simulink model "model_for_lab_2"  (R2022b)
settings: Solver=VariableStepAuto  StartTime=0.0  StopTime=1  RelTol=1e-3
values from neighbouring files (symbols this model uses):
  J = gear_ratio^2 * J_ed    (= 0.0023919264)    [m_for_lab_2.m]
  ke = k_e_static    [m_for_lab_2.m]
  km = ke    [m_for_lab_2.m]
  L = 0.0047    [m_for_lab_2.m]
  R = sum(U .* I) / sum(I.^2)    [m_for_lab_2.m]
  U = str2double(strrep(string(T{:,2}), ',', '.'))    [m_for_lab_2.m]
settings Model: Creator=Eternal_Core  LastModifiedBy=Eternal_Core

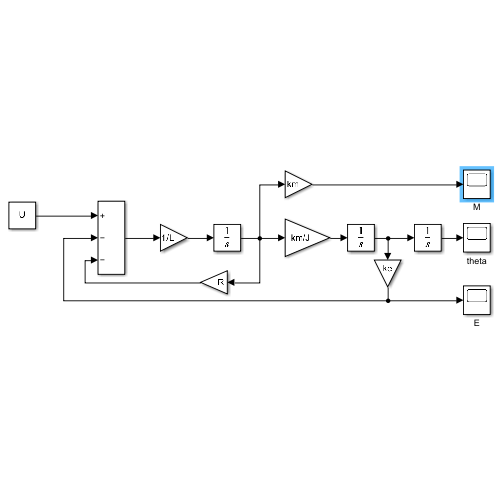
[thumbnail: Simulink's stored preview of the top-level diagram]
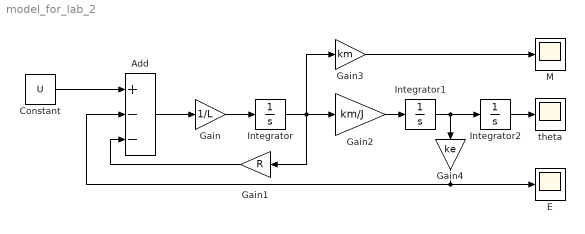
== system model_for_lab_2 ==
  Add : Sum  Inputs=+--
  Constant : Constant  Value=U  SampleTime=-1
  E : Scope
  Gain : Gain  Gain=1/L
  Gain1 : Gain  Gain=R
  Gain2 : Gain  Gain=km/J
  Gain3 : Gain  Gain=km
  Gain4 : Gain  Gain=ke
  Integrator : Integrator
  Integrator1 : Integrator
  Integrator2 : Integrator
  M : Scope
  theta : Scope
  wires:
  Constant/1 -> Add/1
  Add/1 -> Gain/1
  Gain/1 -> Integrator/1
  Integrator/1 -> Gain3/1, Gain1/1, Gain2/1
  Gain1/1 -> Add/3
  Gain3/1 -> M/1
  Gain2/1 -> Integrator1/1
  Integrator1/1 -> Integrator2/1, Gain4/1
  Gain4/1 -> E/1, Add/2
  Integrator2/1 -> theta/1
